simulink model "gm_parallel_prediction_and_cost_function_6phase"  (R2022a)
settings: Solver=FixedStepDiscrete  StartTime=0.0  StopTime=10.0  RelTol=1e-3
undefined symbols (not defined in the file or in its folder): f_c, L_d, L_q, L_x, L_y, p, psi_pm, R_ph
libraries: hdlmdlgenlib x338
(part 4 of 12)

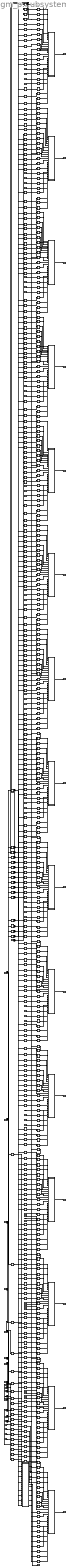
== system gm_parallel_prediction_and_cost_function_6phase/Prediction_and_cost_function/Subsystem ==
  d_phase_voltage_per_switching_state : Inport  OutDataTypeStr=single  PortDimensions=1  SampleTime=1e-08
  q_phase_voltage_per_switching_state : Inport  Port=2  OutDataTypeStr=single  PortDimensions=1  SampleTime=1e-08
  x_phase_voltage_per_switching_state : Inport  Port=3  OutDataTypeStr=single  PortDimensions=1  SampleTime=1e-08
  y_phase_voltage_per_switching_state : Inport  Port=4  OutDataTypeStr=single  PortDimensions=1  SampleTime=1e-08
  d_phase_voltage_per_switching_state1 : Inport  Port=5  OutDataTypeStr=single  PortDimensions=1  SampleTime=1e-08
  q_phase_voltage_per_switching_state1 : Inport  Port=6  OutDataTypeStr=single  PortDimensions=1  SampleTime=1e-08
  x_phase_voltage_per_switching_state1 : Inport  Port=7  OutDataTypeStr=single  PortDimensions=1  SampleTime=1e-08
  y_phase_voltage_per_switching_state1 : Inport  Port=8  OutDataTypeStr=single  PortDimensions=1  SampleTime=1e-08
  d_phase_voltage_per_switching_state2 : Inport  Port=9  OutDataTypeStr=single  PortDimensions=1  SampleTime=1e-08
  q_phase_voltage_per_switching_state2 : Inport  Port=10  OutDataTypeStr=single  PortDimensions=1  SampleTime=1e-08
  x_phase_voltage_per_switching_state2 : Inport  Port=11  OutDataTypeStr=single  PortDimensions=1  SampleTime=1e-08
  y_phase_voltage_per_switching_state2 : Inport  Port=12  OutDataTypeStr=single  PortDimensions=1  SampleTime=1e-08
  d_phase_voltage_per_switching_state3 : Inport  Port=13  OutDataTypeStr=single  PortDimensions=1  SampleTime=1e-08
  q_phase_voltage_per_switching_state3 : Inport  Port=14  OutDataTypeStr=single  PortDimensions=1  SampleTime=1e-08
  x_phase_voltage_per_switching_state3 : Inport  Port=15  OutDataTypeStr=single  PortDimensions=1  SampleTime=1e-08
  y_phase_voltage_per_switching_state3 : Inport  Port=16  OutDataTypeStr=single  PortDimensions=1  SampleTime=1e-08
  d_phase_voltage_per_switching_state4 : Inport  Port=17  OutDataTypeStr=single  PortDimensions=1  SampleTime=1e-08
  q_phase_voltage_per_switching_state4 : Inport  Port=18  OutDataTypeStr=single  PortDimensions=1  SampleTime=1e-08
  x_phase_voltage_per_switching_state4 : Inport  Port=19  OutDataTypeStr=single  PortDimensions=1  SampleTime=1e-08
  y_phase_voltage_per_switching_state4 : Inport  Port=20  OutDataTypeStr=single  PortDimensions=1  SampleTime=1e-08
  d_phase_voltage_per_switching_state5 : Inport  Port=21  OutDataTypeStr=single  PortDimensions=1  SampleTime=1e-08
  q_phase_voltage_per_switching_state5 : Inport  Port=22  OutDataTypeStr=single  PortDimensions=1  SampleTime=1e-08
  x_phase_voltage_per_switching_state5 : Inport  Port=23  OutDataTypeStr=single  PortDimensions=1  SampleTime=1e-08
  y_phase_voltage_per_switching_state5 : Inport  Port=24  OutDataTypeStr=single  PortDimensions=1  SampleTime=1e-08
  d_phase_voltage_per_switching_state6 : Inport  Port=25  OutDataTypeStr=single  PortDimensions=1  SampleTime=1e-08
  q_phase_voltage_per_switching_state6 : Inport  Port=26  OutDataTypeStr=single  PortDimensions=1  SampleTime=1e-08
  x_phase_voltage_per_switching_state6 : Inport  Port=27  OutDataTypeStr=single  PortDimensions=1  SampleTime=1e-08
  y_phase_voltage_per_switching_state6 : Inport  Port=28  OutDataTypeStr=single  PortDimensions=1  SampleTime=1e-08
  d_phase_voltage_per_switching_state7 : Inport  Port=29  OutDataTypeStr=single  PortDimensions=1  SampleTime=1e-08
  q_phase_voltage_per_switching_state7 : Inport  Port=30  OutDataTypeStr=single  PortDimensions=1  SampleTime=1e-08
  x_phase_voltage_per_switching_state7 : Inport  Port=31  OutDataTypeStr=single  PortDimensions=1  SampleTime=1e-08
  y_phase_voltage_per_switching_state7 : Inport  Port=32  OutDataTypeStr=single  PortDimensions=1  SampleTime=1e-08
  d_phase_voltage_per_switching_state8 : Inport  Port=33  OutDataTypeStr=single  PortDimensions=1  SampleTime=1e-08
  q_phase_voltage_per_switching_state8 : Inport  Port=34  OutDataTypeStr=single  PortDimensions=1  SampleTime=1e-08
  x_phase_voltage_per_switching_state8 : Inport  Port=35  OutDataTypeStr=single  PortDimensions=1  SampleTime=1e-08
  y_phase_voltage_per_switching_state8 : Inport  Port=36  OutDataTypeStr=single  PortDimensions=1  SampleTime=1e-08
  d_phase_voltage_per_switching_state9 : Inport  Port=37  OutDataTypeStr=single  PortDimensions=1  SampleTime=1e-08
  q_phase_voltage_per_switching_state9 : Inport  Port=38  OutDataTypeStr=single  PortDimensions=1  SampleTime=1e-08
  x_phase_voltage_per_switching_state9 : Inport  Port=39  OutDataTypeStr=single  PortDimensions=1  SampleTime=1e-08
  y_phase_voltage_per_switching_state9 : Inport  Port=40  OutDataTypeStr=single  PortDimensions=1  SampleTime=1e-08
  d_phase_voltage_per_switching_state10 : Inport  Port=41  OutDataTypeStr=single  PortDimensions=1  SampleTime=1e-08
  q_phase_voltage_per_switching_state10 : Inport  Port=42  OutDataTypeStr=single  PortDimensions=1  SampleTime=1e-08
  x_phase_voltage_per_switching_state10 : Inport  Port=43  OutDataTypeStr=single  PortDimensions=1  SampleTime=1e-08
  y_phase_voltage_per_switching_state10 : Inport  Port=44  OutDataTypeStr=single  PortDimensions=1  SampleTime=1e-08
  d_phase_voltage_per_switching_state11 : Inport  Port=45  OutDataTypeStr=single  PortDimensions=1  SampleTime=1e-08
  q_phase_voltage_per_switching_state11 : Inport  Port=46  OutDataTypeStr=single  PortDimensions=1  SampleTime=1e-08
  x_phase_voltage_per_switching_state11 : Inport  Port=47  OutDataTypeStr=single  PortDimensions=1  SampleTime=1e-08
  y_phase_voltage_per_switching_state11 : Inport  Port=48  OutDataTypeStr=single  PortDimensions=1  SampleTime=1e-08
  d_phase_voltage_per_switching_state12 : Inport  Port=49  OutDataTypeStr=single  PortDimensions=1  SampleTime=1e-08
  q_phase_voltage_per_switching_state12 : Inport  Port=50  OutDataTypeStr=single  PortDimensions=1  SampleTime=1e-08
  x_phase_voltage_per_switching_state12 : Inport  Port=51  OutDataTypeStr=single  PortDimensions=1  SampleTime=1e-08
  y_phase_voltage_per_switching_state12 : Inport  Port=52  OutDataTypeStr=single  PortDimensions=1  SampleTime=1e-08
  d_phase_voltage_per_switching_state13 : Inport  Port=53  OutDataTypeStr=single  PortDimensions=1  SampleTime=1e-08
  q_phase_voltage_per_switching_state13 : Inport  Port=54  OutDataTypeStr=single  PortDimensions=1  SampleTime=1e-08
  x_phase_voltage_per_switching_state13 : Inport  Port=55  OutDataTypeStr=single  PortDimensions=1  SampleTime=1e-08
  y_phase_voltage_per_switching_state13 : Inport  Port=56  OutDataTypeStr=single  PortDimensions=1  SampleTime=1e-08
  d_phase_voltage_per_switching_state14 : Inport  Port=57  OutDataTypeStr=single  PortDimensions=1  SampleTime=1e-08
  q_phase_voltage_per_switching_state14 : Inport  Port=58  OutDataTypeStr=single  PortDimensions=1  SampleTime=1e-08
  x_phase_voltage_per_switching_state14 : Inport  Port=59  OutDataTypeStr=single  PortDimensions=1  SampleTime=1e-08
  y_phase_voltage_per_switching_state14 : Inport  Port=60  OutDataTypeStr=single  PortDimensions=1  SampleTime=1e-08
  SampleTime_div_Ld15 : Inport  Port=61  OutDataTypeStr=single  PortDimensions=1  SampleTime=1e-08
  SampleTime_div_Lq15 : Inport  Port=62  OutDataTypeStr=single  PortDimensions=1  SampleTime=1e-08
  SampleTime_div_Lx15 : Inport  Port=63  OutDataTypeStr=single  PortDimensions=1  SampleTime=1e-08
  SampleTime_div_Ly15 : Inport  Port=64  OutDataTypeStr=single  PortDimensions=1  SampleTime=1e-08
  id_k_16 : Inport  Port=65  OutDataTypeStr=single  PortDimensions=1  SampleTime=1e-08
  iq_k_16 : Inport  Port=66  OutDataTypeStr=single  PortDimensions=1  SampleTime=1e-08
  ix_k_16 : Inport  Port=67  OutDataTypeStr=single  PortDimensions=1  SampleTime=1e-08
  iy_k_16 : Inport  Port=68  OutDataTypeStr=single  PortDimensions=1  SampleTime=1e-08
  Rs15 : Inport  Port=69  OutDataTypeStr=single  PortDimensions=1  SampleTime=1e-08
  omega_el15 : Inport  Port=70  OutDataTypeStr=single  PortDimensions=1  SampleTime=1e-08
  Lq15 : Inport  Port=71  OutDataTypeStr=single  PortDimensions=1  SampleTime=1e-08
  Ld15 : Inport  Port=72  OutDataTypeStr=single  PortDimensions=1  SampleTime=1e-08
  psiPM15 : Inport  Port=73  OutDataTypeStr=single  PortDimensions=1  SampleTime=1e-08
  d_phase_voltage_per_switching_state15 : Inport  Port=74  OutDataTypeStr=single  PortDimensions=1  SampleTime=1e-08
  q_phase_voltage_per_switching_state15 : Inport  Port=75  OutDataTypeStr=single  PortDimensions=1  SampleTime=1e-08
  x_phase_voltage_per_switching_state15 : Inport  Port=76  OutDataTypeStr=single  PortDimensions=1  SampleTime=1e-08
  y_phase_voltage_per_switching_state15 : Inport  Port=77  OutDataTypeStr=single  PortDimensions=1  SampleTime=1e-08
  id_ref15 : Inport  Port=78  OutDataTypeStr=single  PortDimensions=1  SampleTime=1e-08
  iq_ref15 : Inport  Port=79  OutDataTypeStr=single  PortDimensions=1  SampleTime=1e-08
  ix_ref15 : Inport  Port=80  OutDataTypeStr=single  PortDimensions=1  SampleTime=1e-08
  iy_ref15 : Inport  Port=81  OutDataTypeStr=single  PortDimensions=1  SampleTime=1e-08
  From{,1..254} (255 alike) : hdlmdlgenlib/Buffer
      settings: SourceProductBaseCode=SL
  Goto{,1..16} (17 alike) : hdlmdlgenlib/Buffer
      settings: SourceProductBaseCode=SL
  MATLAB Function : Subsystem
  MATLAB Function1 : Subsystem
  MATLAB Function10 : Subsystem
  MATLAB Function11 : Subsystem
  MATLAB Function12 : Subsystem
  MATLAB Function13 : Subsystem
  MATLAB Function14 : Subsystem
  MATLAB Function15 : Subsystem
  MATLAB Function2 : Subsystem
  MATLAB Function3 : Subsystem
  MATLAB Function4 : Subsystem
  MATLAB Function5 : Subsystem
  MATLAB Function6 : Subsystem
  MATLAB Function7 : Subsystem
  MATLAB Function8 : Subsystem
  MATLAB Function9 : Subsystem
  delayMatch{,1..3,8..11,16..23,28..31,36..43,48..51,56..63,68..71,76..83,88..91,96..103,108..111,116..123,128..131,136..143,148..151,156..163,168..171,176..183,188..191,196..203,208..211,216..223,228..231,236..243,248..251,256..263,268..271,276..283,288..291,296..303,308..311,316..319} (192 alike) : Delay  DelayLength=double(12)  InitialCondition=0  SampleTime=1e-08
  delayMatch{4..7,12..15,24..27,32..35,44..47,52..55,64..67,72..75,84..87,92..95,104..107,112..115,124..127,132..135,144..147,152..155,164..167,172..175,184..187,192..195,204..207,212..215,224..227,232..235,244..247,252..255,264..267,272..275,284..287,292..295,304..307,312..315} (128 alike) : Delay  DelayLength=double(6)  InitialCondition=0  SampleTime=1e-08
  J : Outport  SampleTime=1e-08
  J1 : Outport  Port=2  SampleTime=1e-08
  J2 : Outport  Port=3  SampleTime=1e-08
  J3 : Outport  Port=4  SampleTime=1e-08
  J4 : Outport  Port=5  SampleTime=1e-08
  J5 : Outport  Port=6  SampleTime=1e-08
  J6 : Outport  Port=7  SampleTime=1e-08
  J7 : Outport  Port=8  SampleTime=1e-08
  J8 : Outport  Port=9  SampleTime=1e-08
  J9 : Outport  Port=10  SampleTime=1e-08
  J10 : Outport  Port=11  SampleTime=1e-08
  J11 : Outport  Port=12  SampleTime=1e-08
  J12 : Outport  Port=13  SampleTime=1e-08
  J13 : Outport  Port=14  SampleTime=1e-08
  J14 : Outport  Port=15  SampleTime=1e-08
  J15 : Outport  Port=16  SampleTime=1e-08
  wires:
  delayMatch280/1 -> MATLAB Function1/1(SampleTime_div_Ld)
  delayMatch260/1 -> MATLAB Function2/1(SampleTime_div_Ld)
  delayMatch80/1 -> MATLAB Function11/1(SampleTime_div_Ld)
  delayMatch225/1 -> MATLAB Function4/6(iq_k_1)
  delayMatch226/1 -> MATLAB Function4/7(ix_k_1)
  delayMatch227/1 -> MATLAB Function4/8(iy_k_1)
  delayMatch228/1 -> MATLAB Function4/9(Rs)
  From104/1 -> MATLAB Function4/10(omega_el)
  delayMatch229/1 -> MATLAB Function4/11(Lq)
  delayMatch230/1 -> MATLAB Function4/12(Ld)
  delayMatch231/1 -> MATLAB Function4/13(psiPM)
  delayMatch236/1 -> MATLAB Function4/18(id_ref)
  delayMatch237/1 -> MATLAB Function4/19(iq_ref)
  delayMatch60/1 -> MATLAB Function12/1(SampleTime_div_Ld)
  delayMatch238/1 -> MATLAB Function4/20(ix_ref)
  delayMatch239/1 -> MATLAB Function4/21(iy_ref)
  delayMatch204/1 -> MATLAB Function5/5(id_k_1)
  delayMatch205/1 -> MATLAB Function5/6(iq_k_1)
  delayMatch206/1 -> MATLAB Function5/7(ix_k_1)
  delayMatch207/1 -> MATLAB Function5/8(iy_k_1)
  delayMatch208/1 -> MATLAB Function5/9(Rs)
  From117/1 -> MATLAB Function5/10(omega_el)
  delayMatch209/1 -> MATLAB Function5/11(Lq)
  delayMatch210/1 -> MATLAB Function5/12(Ld)
  delayMatch40/1 -> MATLAB Function13/1(SampleTime_div_Ld)
  delayMatch211/1 -> MATLAB Function5/13(psiPM)
  delayMatch216/1 -> MATLAB Function5/18(id_ref)
  delayMatch217/1 -> MATLAB Function5/19(iq_ref)
  delayMatch218/1 -> MATLAB Function5/20(ix_ref)
  delayMatch219/1 -> MATLAB Function5/21(iy_ref)
  delayMatch184/1 -> MATLAB Function6/5(id_k_1)
  delayMatch185/1 -> MATLAB Function6/6(iq_k_1)
  delayMatch186/1 -> MATLAB Function6/7(ix_k_1)
  delayMatch187/1 -> MATLAB Function6/8(iy_k_1)
  delayMatch188/1 -> MATLAB Function6/9(Rs)
  delayMatch20/1 -> MATLAB Function14/1(SampleTime_div_Ld)
  From130/1 -> MATLAB Function6/10(omega_el)
  delayMatch189/1 -> MATLAB Function6/11(Lq)
  delayMatch190/1 -> MATLAB Function6/12(Ld)
  delayMatch191/1 -> MATLAB Function6/13(psiPM)
  delayMatch196/1 -> MATLAB Function6/18(id_ref)
  delayMatch197/1 -> MATLAB Function6/19(iq_ref)
  delayMatch198/1 -> MATLAB Function6/20(ix_ref)
  delayMatch199/1 -> MATLAB Function6/21(iy_ref)
  delayMatch164/1 -> MATLAB Function7/5(id_k_1)
  delayMatch165/1 -> MATLAB Function7/6(iq_k_1)
  delayMatch/1 -> MATLAB Function15/1(SampleTime_div_Ld)
  delayMatch166/1 -> MATLAB Function7/7(ix_k_1)
  delayMatch167/1 -> MATLAB Function7/8(iy_k_1)
  delayMatch168/1 -> MATLAB Function7/9(Rs)
  From143/1 -> MATLAB Function7/10(omega_el)
  delayMatch169/1 -> MATLAB Function7/11(Lq)
  delayMatch170/1 -> MATLAB Function7/12(Ld)
  delayMatch171/1 -> MATLAB Function7/13(psiPM)
  delayMatch176/1 -> MATLAB Function7/18(id_ref)
  delayMatch177/1 -> MATLAB Function7/19(iq_ref)
  delayMatch178/1 -> MATLAB Function7/20(ix_ref)
  delayMatch281/1 -> MATLAB Function1/2(SampleTime_div_Lq)
  delayMatch179/1 -> MATLAB Function7/21(iy_ref)
  delayMatch144/1 -> MATLAB Function8/5(id_k_1)
  delayMatch145/1 -> MATLAB Function8/6(iq_k_1)
  delayMatch146/1 -> MATLAB Function8/7(ix_k_1)
  delayMatch147/1 -> MATLAB Function8/8(iy_k_1)
  delayMatch148/1 -> MATLAB Function8/9(Rs)
  From156/1 -> MATLAB Function8/10(omega_el)
  delayMatch149/1 -> MATLAB Function8/11(Lq)
  delayMatch150/1 -> MATLAB Function8/12(Ld)
  delayMatch151/1 -> MATLAB Function8/13(psiPM)
  delayMatch261/1 -> MATLAB Function2/2(SampleTime_div_Lq)
  delayMatch156/1 -> MATLAB Function8/18(id_ref)
  delayMatch157/1 -> MATLAB Function8/19(iq_ref)
  delayMatch158/1 -> MATLAB Function8/20(ix_ref)
  delayMatch159/1 -> MATLAB Function8/21(iy_ref)
  delayMatch124/1 -> MATLAB Function9/5(id_k_1)
  delayMatch125/1 -> MATLAB Function9/6(iq_k_1)
  delayMatch126/1 -> MATLAB Function9/7(ix_k_1)
  delayMatch127/1 -> MATLAB Function9/8(iy_k_1)
  delayMatch128/1 -> MATLAB Function9/9(Rs)
  From169/1 -> MATLAB Function9/10(omega_el)
  delayMatch241/1 -> MATLAB Function3/2(SampleTime_div_Lq)
  delayMatch129/1 -> MATLAB Function9/11(Lq)
  delayMatch130/1 -> MATLAB Function9/12(Ld)
  delayMatch131/1 -> MATLAB Function9/13(psiPM)
  delayMatch136/1 -> MATLAB Function9/18(id_ref)
  delayMatch137/1 -> MATLAB Function9/19(iq_ref)
  delayMatch138/1 -> MATLAB Function9/20(ix_ref)
  delayMatch139/1 -> MATLAB Function9/21(iy_ref)
  delayMatch104/1 -> MATLAB Function10/5(id_k_1)
  delayMatch105/1 -> MATLAB Function10/6(iq_k_1)
  delayMatch106/1 -> MATLAB Function10/7(ix_k_1)
  delayMatch221/1 -> MATLAB Function4/2(SampleTime_div_Lq)
  delayMatch107/1 -> MATLAB Function10/8(iy_k_1)
  delayMatch108/1 -> MATLAB Function10/9(Rs)
  From182/1 -> MATLAB Function10/10(omega_el)
  delayMatch109/1 -> MATLAB Function10/11(Lq)
  delayMatch110/1 -> MATLAB Function10/12(Ld)
  delayMatch111/1 -> MATLAB Function10/13(psiPM)
  delayMatch116/1 -> MATLAB Function10/18(id_ref)
  delayMatch117/1 -> MATLAB Function10/19(iq_ref)
  delayMatch118/1 -> MATLAB Function10/20(ix_ref)
  delayMatch119/1 -> MATLAB Function10/21(iy_ref)
  delayMatch201/1 -> MATLAB Function5/2(SampleTime_div_Lq)
  delayMatch84/1 -> MATLAB Function11/5(id_k_1)
  delayMatch85/1 -> MATLAB Function11/6(iq_k_1)
  delayMatch86/1 -> MATLAB Function11/7(ix_k_1)
  delayMatch87/1 -> MATLAB Function11/8(iy_k_1)
  delayMatch88/1 -> MATLAB Function11/9(Rs)
  From195/1 -> MATLAB Function11/10(omega_el)
  delayMatch89/1 -> MATLAB Function11/11(Lq)
  delayMatch90/1 -> MATLAB Function11/12(Ld)
  delayMatch91/1 -> MATLAB Function11/13(psiPM)
  delayMatch96/1 -> MATLAB Function11/18(id_ref)
  delayMatch240/1 -> MATLAB Function3/1(SampleTime_div_Ld)
  delayMatch181/1 -> MATLAB Function6/2(SampleTime_div_Lq)
  delayMatch97/1 -> MATLAB Function11/19(iq_ref)
  delayMatch98/1 -> MATLAB Function11/20(ix_ref)
  delayMatch99/1 -> MATLAB Function11/21(iy_ref)
  delayMatch64/1 -> MATLAB Function12/5(id_k_1)
  delayMatch65/1 -> MATLAB Function12/6(iq_k_1)
  delayMatch66/1 -> MATLAB Function12/7(ix_k_1)
  delayMatch67/1 -> MATLAB Function12/8(iy_k_1)
  delayMatch68/1 -> MATLAB Function12/9(Rs)
  From208/1 -> MATLAB Function12/10(omega_el)
  delayMatch69/1 -> MATLAB Function12/11(Lq)
  delayMatch161/1 -> MATLAB Function7/2(SampleTime_div_Lq)
  delayMatch70/1 -> MATLAB Function12/12(Ld)
  delayMatch71/1 -> MATLAB Function12/13(psiPM)
  delayMatch76/1 -> MATLAB Function12/18(id_ref)
  delayMatch77/1 -> MATLAB Function12/19(iq_ref)
  delayMatch78/1 -> MATLAB Function12/20(ix_ref)
  delayMatch79/1 -> MATLAB Function12/21(iy_ref)
  delayMatch44/1 -> MATLAB Function13/5(id_k_1)
  delayMatch45/1 -> MATLAB Function13/6(iq_k_1)
  delayMatch46/1 -> MATLAB Function13/7(ix_k_1)
  delayMatch47/1 -> MATLAB Function13/8(iy_k_1)
  delayMatch141/1 -> MATLAB Function8/2(SampleTime_div_Lq)
  delayMatch48/1 -> MATLAB Function13/9(Rs)
  From221/1 -> MATLAB Function13/10(omega_el)
  delayMatch49/1 -> MATLAB Function13/11(Lq)
  delayMatch50/1 -> MATLAB Function13/12(Ld)
  delayMatch51/1 -> MATLAB Function13/13(psiPM)
  delayMatch56/1 -> MATLAB Function13/18(id_ref)
  delayMatch57/1 -> MATLAB Function13/19(iq_ref)
  delayMatch58/1 -> MATLAB Function13/20(ix_ref)
  delayMatch59/1 -> MATLAB Function13/21(iy_ref)
  delayMatch24/1 -> MATLAB Function14/5(id_k_1)
  delayMatch121/1 -> MATLAB Function9/2(SampleTime_div_Lq)
  delayMatch25/1 -> MATLAB Function14/6(iq_k_1)
  delayMatch26/1 -> MATLAB Function14/7(ix_k_1)
  delayMatch27/1 -> MATLAB Function14/8(iy_k_1)
  delayMatch28/1 -> MATLAB Function14/9(Rs)
  From234/1 -> MATLAB Function14/10(omega_el)
  delayMatch29/1 -> MATLAB Function14/11(Lq)
  delayMatch30/1 -> MATLAB Function14/12(Ld)
  delayMatch31/1 -> MATLAB Function14/13(psiPM)
  delayMatch36/1 -> MATLAB Function14/18(id_ref)
  delayMatch37/1 -> MATLAB Function14/19(iq_ref)
  delayMatch101/1 -> MATLAB Function10/2(SampleTime_div_Lq)
  delayMatch38/1 -> MATLAB Function14/20(ix_ref)
  delayMatch39/1 -> MATLAB Function14/21(iy_ref)
  delayMatch4/1 -> MATLAB Function15/5(id_k_1)
  delayMatch5/1 -> MATLAB Function15/6(iq_k_1)
  delayMatch6/1 -> MATLAB Function15/7(ix_k_1)
  delayMatch7/1 -> MATLAB Function15/8(iy_k_1)
  delayMatch8/1 -> MATLAB Function15/9(Rs)
  From247/1 -> MATLAB Function15/10(omega_el)
  delayMatch9/1 -> MATLAB Function15/11(Lq)
  delayMatch10/1 -> MATLAB Function15/12(Ld)
  delayMatch81/1 -> MATLAB Function11/2(SampleTime_div_Lq)
  delayMatch11/1 -> MATLAB Function15/13(psiPM)
  delayMatch16/1 -> MATLAB Function15/18(id_ref)
  delayMatch17/1 -> MATLAB Function15/19(iq_ref)
  delayMatch18/1 -> MATLAB Function15/20(ix_ref)
  delayMatch19/1 -> MATLAB Function15/21(iy_ref)
  delayMatch61/1 -> MATLAB Function12/2(SampleTime_div_Lq)
  delayMatch41/1 -> MATLAB Function13/2(SampleTime_div_Lq)
  delayMatch21/1 -> MATLAB Function14/2(SampleTime_div_Lq)
  delayMatch1/1 -> MATLAB Function15/2(SampleTime_div_Lq)
  delayMatch220/1 -> MATLAB Function4/1(SampleTime_div_Ld)
  delayMatch282/1 -> MATLAB Function1/3(SampleTime_div_Lx)
  delayMatch262/1 -> MATLAB Function2/3(SampleTime_div_Lx)
  delayMatch242/1 -> MATLAB Function3/3(SampleTime_div_Lx)
  delayMatch222/1 -> MATLAB Function4/3(SampleTime_div_Lx)
  delayMatch202/1 -> MATLAB Function5/3(SampleTime_div_Lx)
  delayMatch182/1 -> MATLAB Function6/3(SampleTime_div_Lx)
  delayMatch162/1 -> MATLAB Function7/3(SampleTime_div_Lx)
  delayMatch142/1 -> MATLAB Function8/3(SampleTime_div_Lx)
  delayMatch122/1 -> MATLAB Function9/3(SampleTime_div_Lx)
  delayMatch102/1 -> MATLAB Function10/3(SampleTime_div_Lx)
  delayMatch200/1 -> MATLAB Function5/1(SampleTime_div_Ld)
  delayMatch82/1 -> MATLAB Function11/3(SampleTime_div_Lx)
  delayMatch62/1 -> MATLAB Function12/3(SampleTime_div_Lx)
  delayMatch42/1 -> MATLAB Function13/3(SampleTime_div_Lx)
  delayMatch22/1 -> MATLAB Function14/3(SampleTime_div_Lx)
  delayMatch2/1 -> MATLAB Function15/3(SampleTime_div_Lx)
  delayMatch283/1 -> MATLAB Function1/4(SampleTime_div_Ly)
  delayMatch263/1 -> MATLAB Function2/4(SampleTime_div_Ly)
  delayMatch243/1 -> MATLAB Function3/4(SampleTime_div_Ly)
  delayMatch223/1 -> MATLAB Function4/4(SampleTime_div_Ly)
  delayMatch203/1 -> MATLAB Function5/4(SampleTime_div_Ly)
  delayMatch180/1 -> MATLAB Function6/1(SampleTime_div_Ld)
  delayMatch183/1 -> MATLAB Function6/4(SampleTime_div_Ly)
  delayMatch163/1 -> MATLAB Function7/4(SampleTime_div_Ly)
  delayMatch143/1 -> MATLAB Function8/4(SampleTime_div_Ly)
  delayMatch123/1 -> MATLAB Function9/4(SampleTime_div_Ly)
  delayMatch103/1 -> MATLAB Function10/4(SampleTime_div_Ly)
  delayMatch83/1 -> MATLAB Function11/4(SampleTime_div_Ly)
  delayMatch63/1 -> MATLAB Function12/4(SampleTime_div_Ly)
  delayMatch43/1 -> MATLAB Function13/4(SampleTime_div_Ly)
  delayMatch23/1 -> MATLAB Function14/4(SampleTime_div_Ly)
  delayMatch3/1 -> MATLAB Function15/4(SampleTime_div_Ly)
  delayMatch160/1 -> MATLAB Function7/1(SampleTime_div_Ld)
  delayMatch284/1 -> MATLAB Function1/5(id_k_1)
  delayMatch285/1 -> MATLAB Function1/6(iq_k_1)
  delayMatch286/1 -> MATLAB Function1/7(ix_k_1)
  delayMatch287/1 -> MATLAB Function1/8(iy_k_1)
  delayMatch288/1 -> MATLAB Function1/9(Rs)
  From65/1 -> MATLAB Function1/10(omega_el)
  delayMatch289/1 -> MATLAB Function1/11(Lq)
  delayMatch290/1 -> MATLAB Function1/12(Ld)
  delayMatch291/1 -> MATLAB Function1/13(psiPM)
  delayMatch296/1 -> MATLAB Function1/18(id_ref)
  delayMatch140/1 -> MATLAB Function8/1(SampleTime_div_Ld)
  delayMatch297/1 -> MATLAB Function1/19(iq_ref)
  delayMatch298/1 -> MATLAB Function1/20(ix_ref)
  delayMatch299/1 -> MATLAB Function1/21(iy_ref)
  delayMatch264/1 -> MATLAB Function2/5(id_k_1)
  delayMatch265/1 -> MATLAB Function2/6(iq_k_1)
  delayMatch266/1 -> MATLAB Function2/7(ix_k_1)
  delayMatch267/1 -> MATLAB Function2/8(iy_k_1)
  delayMatch268/1 -> MATLAB Function2/9(Rs)
  From78/1 -> MATLAB Function2/10(omega_el)
  delayMatch269/1 -> MATLAB Function2/11(Lq)
  delayMatch120/1 -> MATLAB Function9/1(SampleTime_div_Ld)
  delayMatch270/1 -> MATLAB Function2/12(Ld)
  delayMatch271/1 -> MATLAB Function2/13(psiPM)
  delayMatch276/1 -> MATLAB Function2/18(id_ref)
  delayMatch277/1 -> MATLAB Function2/19(iq_ref)
  delayMatch278/1 -> MATLAB Function2/20(ix_ref)
  delayMatch279/1 -> MATLAB Function2/21(iy_ref)
  delayMatch244/1 -> MATLAB Function3/5(id_k_1)
  delayMatch245/1 -> MATLAB Function3/6(iq_k_1)
  delayMatch246/1 -> MATLAB Function3/7(ix_k_1)
  delayMatch247/1 -> MATLAB Function3/8(iy_k_1)
  delayMatch100/1 -> MATLAB Function10/1(SampleTime_div_Ld)
  delayMatch248/1 -> MATLAB Function3/9(Rs)
  From91/1 -> MATLAB Function3/10(omega_el)
  delayMatch249/1 -> MATLAB Function3/11(Lq)
  delayMatch250/1 -> MATLAB Function3/12(Ld)
  delayMatch251/1 -> MATLAB Function3/13(psiPM)
  delayMatch256/1 -> MATLAB Function3/18(id_ref)
  delayMatch257/1 -> MATLAB Function3/19(iq_ref)
  delayMatch258/1 -> MATLAB Function3/20(ix_ref)
  delayMatch259/1 -> MATLAB Function3/21(iy_ref)
  delayMatch224/1 -> MATLAB Function4/5(id_k_1)
  MATLAB Function/1(J) -> J15/1
  MATLAB Function1/1(J) -> J14/1
  MATLAB Function10/1(J) -> J5/1
  MATLAB Function11/1(J) -> J4/1
  MATLAB Function12/1(J) -> J3/1
  MATLAB Function13/1(J) -> J2/1
  MATLAB Function14/1(J) -> J1/1
  MATLAB Function15/1(J) -> J/1
  MATLAB Function2/1(J) -> J13/1
  MATLAB Function3/1(J) -> J12/1
  MATLAB Function4/1(J) -> J11/1
  MATLAB Function5/1(J) -> J10/1
  MATLAB Function6/1(J) -> J9/1
  MATLAB Function7/1(J) -> J8/1
  MATLAB Function8/1(J) -> J7/1
  MATLAB Function9/1(J) -> J6/1
  Goto/1 -> From9/1, From8/1, From7/1, From6/1, From5/1, From4/1, From3/1, From2/1, From14/1, From13/1, From12/1, From11/1, From10/1, From1/1, From/1
  Goto5/1 -> From87/1, From74/1, From61/1, From243/1, From230/1, From217/1, From204/1, From191/1, From178/1, From165/1, From152/1, From139/1, From126/1, From113/1, From100/1
  Goto6/1 -> From88/1, From75/1, From62/1, From244/1, From231/1, From218/1, From205/1, From192/1, From179/1, From166/1, From153/1, From140/1, From127/1, From114/1, From101/1
  Goto7/1 -> From89/1, From76/1, From63/1, From245/1, From232/1, From219/1, From206/1, From193/1, From180/1, From167/1, From154/1, From141/1, From128/1, From115/1, From102/1
  Goto8/1 -> From90/1, From77/1, From64/1, From246/1, From233/1, From220/1, From207/1, From194/1, From181/1, From168/1, From155/1, From142/1, From129/1, From116/1, From103/1
  Goto9/1 -> From91/1, From78/1, From65/1, From247/1, From234/1, From221/1, From208/1, From195/1, From182/1, From169/1, From156/1, From143/1, From130/1, From117/1, From104/1
  Goto10/1 -> From92/1, From79/1, From66/1, From248/1, From235/1, From222/1, From209/1, From196/1, From183/1, From170/1, From157/1, From144/1, From131/1, From118/1, From105/1
  Goto11/1 -> From93/1, From80/1, From67/1, From249/1, From236/1, From223/1, From210/1, From197/1, From184/1, From171/1, From158/1, From145/1, From132/1, From119/1, From106/1
  Goto12/1 -> From94/1, From81/1, From68/1, From250/1, From237/1, From224/1, From211/1, From198/1, From185/1, From172/1, From159/1, From146/1, From133/1, From120/1, From107/1
  Goto13/1 -> From95/1, From82/1, From69/1, From251/1, From238/1, From225/1, From212/1, From199/1, From186/1, From173/1, From160/1, From147/1, From134/1, From121/1, From108/1
  Goto14/1 -> From96/1, From83/1, From70/1, From252/1, From239/1, From226/1, From213/1, From200/1, From187/1, From174/1, From161/1, From148/1, From135/1, From122/1, From109/1
  Goto15/1 -> From97/1, From84/1, From71/1, From253/1, From240/1, From227/1, From214/1, From201/1, From188/1, From175/1, From162/1, From149/1, From136/1, From123/1, From110/1
  Goto16/1 -> From98/1, From85/1, From72/1, From254/1, From241/1, From228/1, From215/1, From202/1, From189/1, From176/1, From163/1, From150/1, From137/1, From124/1, From111/1
  Goto4/1 -> From99/1, From86/1, From73/1, From60/1, From242/1, From229/1, From216/1, From203/1, From190/1, From177/1, From164/1, From151/1, From138/1, From125/1, From112/1
  Goto1/1 -> From29/1, From28/1, From27/1, From26/1, From25/1, From24/1, From23/1, From22/1, From21/1, From20/1, From19/1, From18/1, From17/1, From16/1, From15/1
  Goto2/1 -> From44/1, From43/1, From42/1, From41/1, From40/1, From39/1, From38/1, From37/1, From36/1, From35/1, From34/1, From33/1, From32/1, From31/1, From30/1
  Goto3/1 -> From59/1, From58/1, From57/1, From56/1, From55/1, From54/1, From53/1, From52/1, From51/1, From50/1, From49/1, From48/1, From47/1, From46/1, From45/1
  delayMatch12/1 -> MATLAB Function15/14(d_phase_voltage_per_switching_state)
  delayMatch13/1 -> MATLAB Function15/15(q_phase_voltage_per_switching_state)
  delayMatch14/1 -> MATLAB Function15/16(x_phase_voltage_per_switching_state)
  delayMatch15/1 -> MATLAB Function15/17(y_phase_voltage_per_switching_state)
  delayMatch32/1 -> MATLAB Function14/14(d_phase_voltage_per_switching_state)
  delayMatch33/1 -> MATLAB Function14/15(q_phase_voltage_per_switching_state)
  delayMatch34/1 -> MATLAB Function14/16(x_phase_voltage_per_switching_state)
  delayMatch35/1 -> MATLAB Function14/17(y_phase_voltage_per_switching_state)
  delayMatch52/1 -> MATLAB Function13/14(d_phase_voltage_per_switching_state)
  delayMatch53/1 -> MATLAB Function13/15(q_phase_voltage_per_switching_state)
  delayMatch54/1 -> MATLAB Function13/16(x_phase_voltage_per_switching_state)
  delayMatch55/1 -> MATLAB Function13/17(y_phase_voltage_per_switching_state)
  delayMatch72/1 -> MATLAB Function12/14(d_phase_voltage_per_switching_state)
  delayMatch73/1 -> MATLAB Function12/15(q_phase_voltage_per_switching_state)
  delayMatch74/1 -> MATLAB Function12/16(x_phase_voltage_per_switching_state)
  delayMatch75/1 -> MATLAB Function12/17(y_phase_voltage_per_switching_state)
  delayMatch92/1 -> MATLAB Function11/14(d_phase_voltage_per_switching_state)
  delayMatch93/1 -> MATLAB Function11/15(q_phase_voltage_per_switching_state)
  delayMatch94/1 -> MATLAB Function11/16(x_phase_voltage_per_switching_state)
  delayMatch95/1 -> MATLAB Function11/17(y_phase_voltage_per_switching_state)
  delayMatch112/1 -> MATLAB Function10/14(d_phase_voltage_per_switching_state)
  delayMatch113/1 -> MATLAB Function10/15(q_phase_voltage_per_switching_state)
  delayMatch114/1 -> MATLAB Function10/16(x_phase_voltage_per_switching_state)
  delayMatch115/1 -> MATLAB Function10/17(y_phase_voltage_per_switching_state)
  delayMatch132/1 -> MATLAB Function9/14(d_phase_voltage_per_switching_state)
  delayMatch133/1 -> MATLAB Function9/15(q_phase_voltage_per_switching_state)
  delayMatch134/1 -> MATLAB Function9/16(x_phase_voltage_per_switching_state)
  delayMatch135/1 -> MATLAB Function9/17(y_phase_voltage_per_switching_state)
  delayMatch152/1 -> MATLAB Function8/14(d_phase_voltage_per_switching_state)
  delayMatch153/1 -> MATLAB Function8/15(q_phase_voltage_per_switching_state)
  delayMatch154/1 -> MATLAB Function8/16(x_phase_voltage_per_switching_state)
  delayMatch155/1 -> MATLAB Function8/17(y_phase_voltage_per_switching_state)
  delayMatch172/1 -> MATLAB Function7/14(d_phase_voltage_per_switching_state)
  delayMatch173/1 -> MATLAB Function7/15(q_phase_voltage_per_switching_state)
  delayMatch174/1 -> MATLAB Function7/16(x_phase_voltage_per_switching_state)
  delayMatch175/1 -> MATLAB Function7/17(y_phase_voltage_per_switching_state)
  delayMatch192/1 -> MATLAB Function6/14(d_phase_voltage_per_switching_state)
  delayMatch193/1 -> MATLAB Function6/15(q_phase_voltage_per_switching_state)
  delayMatch194/1 -> MATLAB Function6/16(x_phase_voltage_per_switching_state)
  delayMatch195/1 -> MATLAB Function6/17(y_phase_voltage_per_switching_state)
  delayMatch212/1 -> MATLAB Function5/14(d_phase_voltage_per_switching_state)
  delayMatch213/1 -> MATLAB Function5/15(q_phase_voltage_per_switching_state)
  delayMatch214/1 -> MATLAB Function5/16(x_phase_voltage_per_switching_state)
  delayMatch215/1 -> MATLAB Function5/17(y_phase_voltage_per_switching_state)
  delayMatch232/1 -> MATLAB Function4/14(d_phase_voltage_per_switching_state)
  delayMatch233/1 -> MATLAB Function4/15(q_phase_voltage_per_switching_state)
  delayMatch234/1 -> MATLAB Function4/16(x_phase_voltage_per_switching_state)
  delayMatch235/1 -> MATLAB Function4/17(y_phase_voltage_per_switching_state)
  delayMatch252/1 -> MATLAB Function3/14(d_phase_voltage_per_switching_state)
  delayMatch253/1 -> MATLAB Function3/15(q_phase_voltage_per_switching_state)
  delayMatch254/1 -> MATLAB Function3/16(x_phase_voltage_per_switching_state)
  delayMatch255/1 -> MATLAB Function3/17(y_phase_voltage_per_switching_state)
  delayMatch272/1 -> MATLAB Function2/14(d_phase_voltage_per_switching_state)
  delayMatch273/1 -> MATLAB Function2/15(q_phase_voltage_per_switching_state)
  delayMatch274/1 -> MATLAB Function2/16(x_phase_voltage_per_switching_state)
  delayMatch275/1 -> MATLAB Function2/17(y_phase_voltage_per_switching_state)
  delayMatch292/1 -> MATLAB Function1/14(d_phase_voltage_per_switching_state)
  delayMatch293/1 -> MATLAB Function1/15(q_phase_voltage_per_switching_state)
  delayMatch294/1 -> MATLAB Function1/16(x_phase_voltage_per_switching_state)
  delayMatch295/1 -> MATLAB Function1/17(y_phase_voltage_per_switching_state)
  delayMatch300/1 -> MATLAB Function/1(SampleTime_div_Ld)
  delayMatch301/1 -> MATLAB Function/2(SampleTime_div_Lq)
  delayMatch302/1 -> MATLAB Function/3(SampleTime_div_Lx)
  delayMatch303/1 -> MATLAB Function/4(SampleTime_div_Ly)
  delayMatch304/1 -> MATLAB Function/5(id_k_1)
  delayMatch305/1 -> MATLAB Function/6(iq_k_1)
  delayMatch306/1 -> MATLAB Function/7(ix_k_1)
  delayMatch307/1 -> MATLAB Function/8(iy_k_1)
  delayMatch308/1 -> MATLAB Function/9(Rs)
  delayMatch309/1 -> MATLAB Function/11(Lq)
  delayMatch310/1 -> MATLAB Function/12(Ld)
  delayMatch311/1 -> MATLAB Function/13(psiPM)
  delayMatch312/1 -> MATLAB Function/14(d_phase_voltage_per_switching_state)
  delayMatch313/1 -> MATLAB Function/15(q_phase_voltage_per_switching_state)
  delayMatch314/1 -> MATLAB Function/16(x_phase_voltage_per_switching_state)
  delayMatch315/1 -> MATLAB Function/17(y_phase_voltage_per_switching_state)
  delayMatch316/1 -> MATLAB Function/18(id_ref)
  delayMatch317/1 -> MATLAB Function/19(iq_ref)
  delayMatch318/1 -> MATLAB Function/20(ix_ref)
  delayMatch319/1 -> MATLAB Function/21(iy_ref)
  From14/1 -> delayMatch/1
  From29/1 -> delayMatch1/1
  From44/1 -> delayMatch2/1
  From59/1 -> delayMatch3/1
  From242/1 -> delayMatch4/1
  From243/1 -> delayMatch5/1
  From244/1 -> delayMatch6/1
  From245/1 -> delayMatch7/1
  From246/1 -> delayMatch8/1
  From248/1 -> delayMatch9/1
  From249/1 -> delayMatch10/1
  From250/1 -> delayMatch11/1
  From251/1 -> delayMatch16/1
  From252/1 -> delayMatch17/1
  From253/1 -> delayMatch18/1
  From254/1 -> delayMatch19/1
  From13/1 -> delayMatch20/1
  From28/1 -> delayMatch21/1
  From43/1 -> delayMatch22/1
  From58/1 -> delayMatch23/1
  From229/1 -> delayMatch24/1
  From230/1 -> delayMatch25/1
  From231/1 -> delayMatch26/1
  From232/1 -> delayMatch27/1
  From233/1 -> delayMatch28/1
  From235/1 -> delayMatch29/1
  From236/1 -> delayMatch30/1
  From237/1 -> delayMatch31/1
  From238/1 -> delayMatch36/1
  From239/1 -> delayMatch37/1
  From240/1 -> delayMatch38/1
  From241/1 -> delayMatch39/1
  From12/1 -> delayMatch40/1
  From27/1 -> delayMatch41/1
  From42/1 -> delayMatch42/1
  From57/1 -> delayMatch43/1
  From216/1 -> delayMatch44/1
  From217/1 -> delayMatch45/1
  From218/1 -> delayMatch46/1
  From219/1 -> delayMatch47/1
  From220/1 -> delayMatch48/1
  From222/1 -> delayMatch49/1
  From223/1 -> delayMatch50/1
  From224/1 -> delayMatch51/1
  From225/1 -> delayMatch56/1
  From226/1 -> delayMatch57/1
  From227/1 -> delayMatch58/1
  From228/1 -> delayMatch59/1
  From11/1 -> delayMatch60/1
  From26/1 -> delayMatch61/1
  From41/1 -> delayMatch62/1
  From56/1 -> delayMatch63/1
  From203/1 -> delayMatch64/1
  From204/1 -> delayMatch65/1
  From205/1 -> delayMatch66/1
  From206/1 -> delayMatch67/1
  From207/1 -> delayMatch68/1
  From209/1 -> delayMatch69/1
  From210/1 -> delayMatch70/1
  From211/1 -> delayMatch71/1
  From212/1 -> delayMatch76/1
  From213/1 -> delayMatch77/1
  From214/1 -> delayMatch78/1
  From215/1 -> delayMatch79/1
  From10/1 -> delayMatch80/1
  From25/1 -> delayMatch81/1
  From40/1 -> delayMatch82/1
  From55/1 -> delayMatch83/1
  From190/1 -> delayMatch84/1
  From191/1 -> delayMatch85/1
  From192/1 -> delayMatch86/1
  From193/1 -> delayMatch87/1
  From194/1 -> delayMatch88/1
  From196/1 -> delayMatch89/1
  From197/1 -> delayMatch90/1
  From198/1 -> delayMatch91/1
  From199/1 -> delayMatch96/1
  From200/1 -> delayMatch97/1
  From201/1 -> delayMatch98/1
  From202/1 -> delayMatch99/1
  From9/1 -> delayMatch100/1
  From24/1 -> delayMatch101/1
  From39/1 -> delayMatch102/1
  From54/1 -> delayMatch103/1
  From177/1 -> delayMatch104/1
  From178/1 -> delayMatch105/1
  From179/1 -> delayMatch106/1
  From180/1 -> delayMatch107/1
  From181/1 -> delayMatch108/1
  From183/1 -> delayMatch109/1
  From184/1 -> delayMatch110/1
  From185/1 -> delayMatch111/1
  From186/1 -> delayMatch116/1
  From187/1 -> delayMatch117/1
  From188/1 -> delayMatch118/1
  From189/1 -> delayMatch119/1
  From8/1 -> delayMatch120/1
  From23/1 -> delayMatch121/1
  From38/1 -> delayMatch122/1
  From53/1 -> delayMatch123/1
  From164/1 -> delayMatch124/1
  From165/1 -> delayMatch125/1
  From166/1 -> delayMatch126/1
  From167/1 -> delayMatch127/1
  From168/1 -> delayMatch128/1
  From170/1 -> delayMatch129/1
  From171/1 -> delayMatch130/1
  From172/1 -> delayMatch131/1
  From173/1 -> delayMatch136/1
  From174/1 -> delayMatch137/1
  From175/1 -> delayMatch138/1
  From176/1 -> delayMatch139/1
  From7/1 -> delayMatch140/1
  From22/1 -> delayMatch141/1
  From37/1 -> delayMatch142/1
  From52/1 -> delayMatch143/1
  From151/1 -> delayMatch144/1
  From152/1 -> delayMatch145/1
  From153/1 -> delayMatch146/1
  From154/1 -> delayMatch147/1
  From155/1 -> delayMatch148/1
  From157/1 -> delayMatch149/1
  From158/1 -> delayMatch150/1
  From159/1 -> delayMatch151/1
  From160/1 -> delayMatch156/1
  From161/1 -> delayMatch157/1
  From162/1 -> delayMatch158/1
  From163/1 -> delayMatch159/1
  From6/1 -> delayMatch160/1
  From21/1 -> delayMatch161/1
  From36/1 -> delayMatch162/1
  From51/1 -> delayMatch163/1
  From138/1 -> delayMatch164/1
  From139/1 -> delayMatch165/1
  From140/1 -> delayMatch166/1
  From141/1 -> delayMatch167/1
  From142/1 -> delayMatch168/1
  From144/1 -> delayMatch169/1
  From145/1 -> delayMatch170/1
  From146/1 -> delayMatch171/1
  From147/1 -> delayMatch176/1
  From148/1 -> delayMatch177/1
  From149/1 -> delayMatch178/1
  From150/1 -> delayMatch179/1
  From5/1 -> delayMatch180/1
  From20/1 -> delayMatch181/1
  From35/1 -> delayMatch182/1
  From50/1 -> delayMatch183/1
  From125/1 -> delayMatch184/1
  From126/1 -> delayMatch185/1
  From127/1 -> delayMatch186/1
  From128/1 -> delayMatch187/1
  From129/1 -> delayMatch188/1
  From131/1 -> delayMatch189/1
  From132/1 -> delayMatch190/1
  From133/1 -> delayMatch191/1
  From134/1 -> delayMatch196/1
  From135/1 -> delayMatch197/1
  From136/1 -> delayMatch198/1
  From137/1 -> delayMatch199/1
  From4/1 -> delayMatch200/1
  From19/1 -> delayMatch201/1
  From34/1 -> delayMatch202/1
  From49/1 -> delayMatch203/1
  From112/1 -> delayMatch204/1
  From113/1 -> delayMatch205/1
  From114/1 -> delayMatch206/1
  From115/1 -> delayMatch207/1
  From116/1 -> delayMatch208/1
  From118/1 -> delayMatch209/1
  From119/1 -> delayMatch210/1
  From120/1 -> delayMatch211/1
  From121/1 -> delayMatch216/1
  From122/1 -> delayMatch217/1
  From123/1 -> delayMatch218/1
  From124/1 -> delayMatch219/1
  From3/1 -> delayMatch220/1
  From18/1 -> delayMatch221/1
  From33/1 -> delayMatch222/1
  From48/1 -> delayMatch223/1
  From99/1 -> delayMatch224/1
  From100/1 -> delayMatch225/1
  From101/1 -> delayMatch226/1
  From102/1 -> delayMatch227/1
  From103/1 -> delayMatch228/1
  From105/1 -> delayMatch229/1
  From106/1 -> delayMatch230/1
  From107/1 -> delayMatch231/1
  From108/1 -> delayMatch236/1
  From109/1 -> delayMatch237/1
  From110/1 -> delayMatch238/1
  From111/1 -> delayMatch239/1
  From2/1 -> delayMatch240/1
  From17/1 -> delayMatch241/1
  From32/1 -> delayMatch242/1
  From47/1 -> delayMatch243/1
  From86/1 -> delayMatch244/1
  From87/1 -> delayMatch245/1
  From88/1 -> delayMatch246/1
  From89/1 -> delayMatch247/1
  From90/1 -> delayMatch248/1
  From92/1 -> delayMatch249/1
  From93/1 -> delayMatch250/1
  From94/1 -> delayMatch251/1
  From95/1 -> delayMatch256/1
  From96/1 -> delayMatch257/1
  From97/1 -> delayMatch258/1
  From98/1 -> delayMatch259/1
  From1/1 -> delayMatch260/1
  From16/1 -> delayMatch261/1
  From31/1 -> delayMatch262/1
  From46/1 -> delayMatch263/1
  From73/1 -> delayMatch264/1
  From74/1 -> delayMatch265/1
  From75/1 -> delayMatch266/1
  From76/1 -> delayMatch267/1
  From77/1 -> delayMatch268/1
  From79/1 -> delayMatch269/1
  From80/1 -> delayMatch270/1
  From81/1 -> delayMatch271/1
  From82/1 -> delayMatch276/1
  From83/1 -> delayMatch277/1
  From84/1 -> delayMatch278/1
  From85/1 -> delayMatch279/1
  From/1 -> delayMatch280/1
  From15/1 -> delayMatch281/1
  From30/1 -> delayMatch282/1
  From45/1 -> delayMatch283/1
  From60/1 -> delayMatch284/1
  From61/1 -> delayMatch285/1
  From62/1 -> delayMatch286/1
  From63/1 -> delayMatch287/1
  From64/1 -> delayMatch288/1
  From66/1 -> delayMatch289/1
  From67/1 -> delayMatch290/1
  From68/1 -> delayMatch291/1
  From69/1 -> delayMatch296/1
  From70/1 -> delayMatch297/1
  From71/1 -> delayMatch298/1
  From72/1 -> delayMatch299/1
  d_phase_voltage_per_switching_state/1 -> delayMatch12/1
  q_phase_voltage_per_switching_state/1 -> delayMatch13/1
  x_phase_voltage_per_switching_state/1 -> delayMatch14/1
  y_phase_voltage_per_switching_state/1 -> delayMatch15/1
  d_phase_voltage_per_switching_state1/1 -> delayMatch32/1
  q_phase_voltage_per_switching_state1/1 -> delayMatch33/1
  x_phase_voltage_per_switching_state1/1 -> delayMatch34/1
  y_phase_voltage_per_switching_state1/1 -> delayMatch35/1
  d_phase_voltage_per_switching_state2/1 -> delayMatch52/1
  q_phase_voltage_per_switching_state2/1 -> delayMatch53/1
  x_phase_voltage_per_switching_state2/1 -> delayMatch54/1
  y_phase_voltage_per_switching_state2/1 -> delayMatch55/1
  d_phase_voltage_per_switching_state3/1 -> delayMatch72/1
  q_phase_voltage_per_switching_state3/1 -> delayMatch73/1
  x_phase_voltage_per_switching_state3/1 -> delayMatch74/1
  y_phase_voltage_per_switching_state3/1 -> delayMatch75/1
  d_phase_voltage_per_switching_state4/1 -> delayMatch92/1
  q_phase_voltage_per_switching_state4/1 -> delayMatch93/1
  x_phase_voltage_per_switching_state4/1 -> delayMatch94/1
  y_phase_voltage_per_switching_state4/1 -> delayMatch95/1
  d_phase_voltage_per_switching_state5/1 -> delayMatch112/1
  q_phase_voltage_per_switching_state5/1 -> delayMatch113/1
  x_phase_voltage_per_switching_state5/1 -> delayMatch114/1
  y_phase_voltage_per_switching_state5/1 -> delayMatch115/1
  d_phase_voltage_per_switching_state6/1 -> delayMatch132/1
  q_phase_voltage_per_switching_state6/1 -> delayMatch133/1
  x_phase_voltage_per_switching_state6/1 -> delayMatch134/1
  y_phase_voltage_per_switching_state6/1 -> delayMatch135/1
  d_phase_voltage_per_switching_state7/1 -> delayMatch152/1
  q_phase_voltage_per_switching_state7/1 -> delayMatch153/1
  x_phase_voltage_per_switching_state7/1 -> delayMatch154/1
  y_phase_voltage_per_switching_state7/1 -> delayMatch155/1
  d_phase_voltage_per_switching_state8/1 -> delayMatch172/1
  q_phase_voltage_per_switching_state8/1 -> delayMatch173/1
  x_phase_voltage_per_switching_state8/1 -> delayMatch174/1
  y_phase_voltage_per_switching_state8/1 -> delayMatch175/1
  d_phase_voltage_per_switching_state9/1 -> delayMatch192/1
  q_phase_voltage_per_switching_state9/1 -> delayMatch193/1
  x_phase_voltage_per_switching_state9/1 -> delayMatch194/1
  y_phase_voltage_per_switching_state9/1 -> delayMatch195/1
  d_phase_voltage_per_switching_state10/1 -> delayMatch212/1
  q_phase_voltage_per_switching_state10/1 -> delayMatch213/1
  x_phase_voltage_per_switching_state10/1 -> delayMatch214/1
  y_phase_voltage_per_switching_state10/1 -> delayMatch215/1
  d_phase_voltage_per_switching_state11/1 -> delayMatch232/1
  q_phase_voltage_per_switching_state11/1 -> delayMatch233/1
  x_phase_voltage_per_switching_state11/1 -> delayMatch234/1
  y_phase_voltage_per_switching_state11/1 -> delayMatch235/1
  d_phase_voltage_per_switching_state12/1 -> delayMatch252/1
  q_phase_voltage_per_switching_state12/1 -> delayMatch253/1
  x_phase_voltage_per_switching_state12/1 -> delayMatch254/1
  y_phase_voltage_per_switching_state12/1 -> delayMatch255/1
  d_phase_voltage_per_switching_state13/1 -> delayMatch272/1
  q_phase_voltage_per_switching_state13/1 -> delayMatch273/1
  x_phase_voltage_per_switching_state13/1 -> delayMatch274/1
  y_phase_voltage_per_switching_state13/1 -> delayMatch275/1
  d_phase_voltage_per_switching_state14/1 -> delayMatch292/1
  q_phase_voltage_per_switching_state14/1 -> delayMatch293/1
  x_phase_voltage_per_switching_state14/1 -> delayMatch294/1
  y_phase_voltage_per_switching_state14/1 -> delayMatch295/1
  SampleTime_div_Ld15/1 -> delayMatch300/1, Goto/1
  SampleTime_div_Lq15/1 -> delayMatch301/1, Goto1/1
  SampleTime_div_Lx15/1 -> delayMatch302/1, Goto2/1
  SampleTime_div_Ly15/1 -> delayMatch303/1, Goto3/1
  id_k_16/1 -> delayMatch304/1, Goto4/1
  iq_k_16/1 -> delayMatch305/1, Goto5/1
  ix_k_16/1 -> delayMatch306/1, Goto6/1
  iy_k_16/1 -> delayMatch307/1, Goto7/1
  Rs15/1 -> delayMatch308/1, Goto8/1
  omega_el15/1 -> Goto9/1, MATLAB Function/10(omega_el)
  Lq15/1 -> delayMatch309/1, Goto10/1
  Ld15/1 -> delayMatch310/1, Goto11/1
  psiPM15/1 -> delayMatch311/1, Goto12/1
  d_phase_voltage_per_switching_state15/1 -> delayMatch312/1
  q_phase_voltage_per_switching_state15/1 -> delayMatch313/1
  x_phase_voltage_per_switching_state15/1 -> delayMatch314/1
  y_phase_voltage_per_switching_state15/1 -> delayMatch315/1
  id_ref15/1 -> delayMatch316/1, Goto13/1
  iq_ref15/1 -> delayMatch317/1, Goto14/1
  ix_ref15/1 -> delayMatch318/1, Goto15/1
  iy_ref15/1 -> delayMatch319/1, Goto16/1

== system gm_parallel_prediction_and_cost_function_6phase/Prediction_and_cost_function/Detect Rise Positive/Positive ==
  u : Inport  OutDataTypeStr=boolean  SampleTime=1e-08
  Compare : RelationalOperator  Operator=>  OutDataTypeStr=boolean  ZeroCross=off
  Constant : Constant  DisableCoverage=on  Value=0  OutDataTypeStr=Inherit: Inherit via back propagation  SampleTime=-1  PreserveConstantTs=on
  y : Outport  SampleTime=1e-08
  wires:
  Compare/1 -> y/1
  Constant/1 -> Compare/2
  u/1 -> Compare/1

== system gm_parallel_prediction_and_cost_function_6phase/Prediction_and_cost_function/Detect Rise Positive1/Positive ==
  u : Inport  OutDataTypeStr=boolean  SampleTime=1e-08
  Compare : RelationalOperator  Operator=>  OutDataTypeStr=boolean  ZeroCross=off
  Constant : Constant  DisableCoverage=on  Value=0  OutDataTypeStr=Inherit: Inherit via back propagation  SampleTime=-1  PreserveConstantTs=on
  y : Outport  SampleTime=1e-08
  wires:
  Compare/1 -> y/1
  Constant/1 -> Compare/2
  u/1 -> Compare/1

== system gm_parallel_prediction_and_cost_function_6phase/Prediction_and_cost_function/Detect Rise Positive2/Positive ==
  u : Inport  OutDataTypeStr=boolean  SampleTime=1e-08
  Compare : RelationalOperator  Operator=>  OutDataTypeStr=boolean  ZeroCross=off
  Constant : Constant  DisableCoverage=on  Value=0  OutDataTypeStr=Inherit: Inherit via back propagation  SampleTime=-1  PreserveConstantTs=on
  y : Outport  SampleTime=1e-08
  wires:
  Compare/1 -> y/1
  Constant/1 -> Compare/2
  u/1 -> Compare/1
